simulink model "SimLaserGame"  (R2020a)
settings: Solver=VariableStepAuto  StartTime=0.0  StopTime=0.1  RelTol=1e-3
values from neighbouring files (symbols this model uses):
  den = [1.7483*10^(-23) 7.6663*10^(-18) 1.162*10^(-11) 3.0332*10^(-6) 1]    [ScriptLaserGame.m]
  Fsin1 = 85000    [ScriptLaserGame.m]
  Fsin2 = 90000    [ScriptLaserGame.m]
  Fsin3 = 94986.8    [ScriptLaserGame.m]
  Fsin4 = 100000    [ScriptLaserGame.m]
  Fsin5 = 115015.9    [ScriptLaserGame.m]
  Fsin6 = 120000    [ScriptLaserGame.m]
  Te = T/M    (= 0.0078125)    [ScriptDFT.m]    (also in ScriptLaserGame.m = 3.125e-06)
settings Model: Creator=benyahia  LastModifiedBy=benyahia

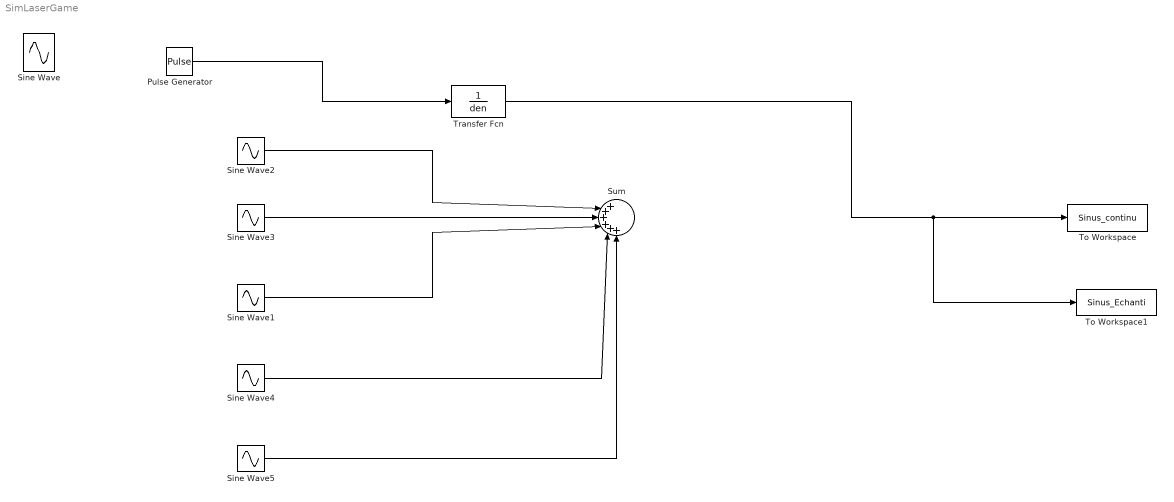
== system SimLaserGame ==
  Pulse Generator : DiscretePulseGenerator  PulseType=Time based  Period=1/Fsin1  PulseWidth=50
  Sine Wave : Sin  Frequency=2*pi*Fsin1  SampleTime=0
  Sine Wave1 : Sin  Frequency=2*pi*Fsin4  SampleTime=0
  Sine Wave2 : Sin  Frequency=2*pi*Fsin2  SampleTime=0
  Sine Wave3 : Sin  Frequency=2*pi*Fsin3  SampleTime=0
  Sine Wave4 : Sin  Frequency=2*pi*Fsin5  SampleTime=0
  Sine Wave5 : Sin  Frequency=2*pi*Fsin6  SampleTime=0
  Sum : Sum  Inputs=|++++++
  To Workspace : ToWorkspace  VariableName=Sinus_continu  SaveFormat=Timeseries  SampleTime=Te/100
  To Workspace1 : ToWorkspace  VariableName=Sinus_Echanti  SaveFormat=Timeseries  SampleTime=Te
  Transfer Fcn : TransferFcn  Denominator=den
  wires:
  Sine Wave2/1 -> Sum/2
  Sine Wave3/1 -> Sum/3
  Sine Wave1/1 -> Sum/4
  Sine Wave4/1 -> Sum/5
  Sine Wave5/1 -> Sum/6
  Transfer Fcn/1 -> To Workspace1/1, To Workspace/1
  Pulse Generator/1 -> Transfer Fcn/1
